simulink model "automata_learning"  (R2022a)
(part 4 of 10)

(exp(0.08277370035648346 * x1 + 0.14355190098285675 * x2 + 0.11031784117221832) - 1.0) / (exp(0.08277370035648346 * x1 + 0.14355190098285675 * x2 + 0.11031784117221832) + 1.0) - 0.17225147783756256 * (exp(0.9740955233573914 * x1 - 0.5740582346916199 * x2 + 0.584020733833313) - 1.0) / (exp(0.9740955233573914 * x1 - 0.5740582346916199 * x2 + 0.584020733833313) + 1.0) - 0.14975093305110931 * (exp(0.2844334542751312 * x1 - 0.20399335026741028 * x2 + 0.39677372574806213) - 1.0) / (exp(0.2844334542751312 * x1 - 0.20399335026741028 * x2 + 0.39677372574806213) + 1.0) - 0.6673128008842468 * (exp(0.12507730722427368 * x1 + 0.22762612998485565 * x2 + 0.3865107297897339) - 1.0) / (exp(0.12507730722427368 * x1 + 0.22762612998485565 * x2 + 0.3865107297897339) + 1.0) + 0.31276842951774597 * (exp(0.5199534296989441 * x1 - 0.738328218460083 * x2 + 0.49007365107536316) - 1.0) / (exp(0.5199534296989441 * x1 - 0.738328218460083 * x2 + 0.49007365107536316) + 1.0) - 0.4881001114845276 * (exp(0.8014535307884216 * x1 - 0.28345319628715515 * x2 + 0.22281718254089355) - 1.0) / (exp(0.8014535307884216 * x1 - 0.28345319628715515 * x2 + 0.22281718254089355) + 1.0) + 0.46977734565734863 * (exp(1.577635645866394 * x1 + 0.23506608605384827 * x2 - 0.06673777848482132) - 1.0) / (exp(1.577635645866394 * x1 + 0.23506608605384827 * x2 - 0.06673777848482132) + 1.0) + 0.3694143295288086 * (exp(0.9763611555099487 * x1 + 1.2415034770965576 * x2 - 0.16854457557201385) - 1.0) / (exp(0.9763611555099487 * x1 + 1.2415034770965576 * x2 - 0.16854457557201385) + 1.0) + 0.12421704083681107 * (exp(0.9488367438316345 * x2 - 0.4073374271392822 * x1 + 0.07838433980941772) - 1.0) / (exp(0.9488367438316345 * x2 - 0.4073374271392822 * x1 + 0.07838433980941772) + 1.0) + 0.6204631328582764 * (exp(1.727070927619934 * x1 + 0.877204418182373 * x2 + 0.7861019372940063) - 1.0) / (exp(1.727070927619934 * x1 + 0.877204418182373 * x2 + 0.7861019372940063) + 1.0) + 2.2496016025543213 * (exp(0.0031111659482121468 * x2 - 1.920979619026184 * x1 + 1.6593092679977417) - 1.0) / (exp(0.0031111659482121468 * x2 - 1.920979619026184 * x1 + 1.6593092679977417) + 1.0) + 0.0063673099502921104) + 1.0) - 0.01678931713104248 * (exp(0.025701038539409637 * (exp(0.2574288547039032 * x2 - 0.6871621012687683 * x1 + 0.5600507855415344) - 1.0) / (exp(0.2574288547039032 * x2 - 0.6871621012687683 * x1 + 0.5600507855415344) + 1.0) - 0.6211979985237122 * (exp(0.28132522106170654 * x2 - 0.539489209651947 * x1 + 0.6009179949760437) - 1.0) / (exp(0.28132522106170654 * x2 - 0.539489209651947 * x1 + 0.6009179949760437) + 1.0) - 0.07466983050107956 * (exp(0.23744763433933258 * x2 - 0.9225135445594788 * x1 + 0.3782052993774414) - 1.0) / (exp(0.23744763433933258 * x2 - 0.9225135445594788 * x1 + 0.3782052993774414) + 1.0) - 0.6362066268920898 * (exp(0.5844773054122925 * x2 - 0.2779636085033417 * x1 + 0.6274034380912781) - 1.0) / (exp(0.5844773054122925 * x2 - 0.2779636085033417 * x1 + 0.6274034380912781) + 1.0) + 0.18158797919750214 * (exp(0.18866761028766632 * x1 + 0.25410085916519165 * x2 + 0.5283621549606323) - 1.0) / (exp(0.18866761028766632 * x1 + 0.25410085916519165 * x2 + 0.5283621549606323) + 1.0) + 0.7426992654800415 * (exp(1.1490525007247925 * x1 - 0.646297037601471 * x2 + 0.6117565035820007) - 1.0) / (exp(1.1490525007247925 * x1 - 0.646297037601471 * x2 + 0.6117565035820007) + 1.0) + 0.16969242691993713 * (exp(0.20323987305164337 * x1 + 0.5146556496620178 * x2 + 0.6071406602859497) - 1.0) / (exp(0.20323987305164337 * x1 + 0.5146556496620178 * x2 + 0.6071406602859497) + 1.0) + 0.10171923041343689 * (exp(0.5478074550628662 * x1 + 0.33825451135635376 * x2 + 0.42206645011901855) - 1.0) / (exp(0.5478074550628662 * x1 + 0.33825451135635376 * x2 + 0.42206645011901855) + 1.0) - 0.7393468022346497 * (exp(1.1907950639724731 * x1 + 0.3422628939151764 * x2 - 0.10066080093383789) - 1.0) / (exp(1.1907950639724731 * x1 + 0.3422628939151764 * x2 - 0.10066080093383789) + 1.0) + 0.05626780539751053 * (exp(0.08277370035648346 * x1 + 0.14355190098285675 * x2 + 0.11031784117221832) - 1.0) / (exp(0.08277370035648346 * x1 + 0.14355190098285675 * x2 + 0.11031784117221832) + 1.0) + 0.754966676235199 * (exp(0.9740955233573914 * x1 - 0.5740582346916199 * x2 + 0.584020733833313) - 1.0) / (exp(0.9740955233573914 * x1 - 0.5740582346916199 * x2 + 0.584020733833313) + 1.0) + 0.7143430113792419 * (exp(0.2844334542751312 * x1 - 0.20399335026741028 * x2 + 0.39677372574806213) - 1.0) / (exp(0.2844334542751312 * x1 - 0.20399335026741028 * x2 + 0.39677372574806213) + 1.0) + 0.6644455790519714 * (exp(0.12507730722427368 * x1 + 0.22762612998485565 * x2 + 0.3865107297897339) - 1.0) / (exp(0.12507730722427368 * x1 + 0.22762612998485565 * x2 + 0.3865107297897339) + 1.0) - 0.20606382191181183 * (exp(0.5199534296989441 * x1 - 0.738328218460083 * x2 + 0.49007365107536316) - 1.0) / (exp(0.5199534296989441 * x1 - 0.738328218460083 * x2 + 0.49007365107536316) + 1.0) + 0.4566824436187744 * (exp(0.8014535307884216 * x1 - 0.28345319628715515 * x2 + 0.22281718254089355) - 1.0) / (exp(0.8014535307884216 * x1 - 0.28345319628715515 * x2 + 0.22281718254089355) + 1.0) - 0.7963041067123413 * (exp(1.577635645866394 * x1 + 0.23506608605384827 * x2 - 0.06673777848482132) - 1.0) / (exp(1.577635645866394 * x1 + 0.23506608605384827 * x2 - 0.06673777848482132) + 1.0) - 0.2628166675567627 * (exp(0.9763611555099487 * x1 + 1.2415034770965576 * x2 - 0.16854457557201385) - 1.0) / (exp(0.9763611555099487 * x1 + 1.2415034770965576 * x2 - 0.16854457557201385) + 1.0) + 0.245744988322258 * (exp(0.9488367438316345 * x2 - 0.4073374271392822 * x1 + 0.07838433980941772) - 1.0) / (exp(0.9488367438316345 * x2 - 0.4073374271392822 * x1 + 0.07838433980941772) + 1.0) + 0.47640275955200195 * (exp(1.727070927619934 * x1 + 0.877204418182373 * x2 + 0.7861019372940063) - 1.0) / (exp(1.727070927619934 * x1 + 0.877204418182373 * x2 + 0.7861019372940063) + 1.0) + 0.15228034555912018 * (exp(0.0031111659482121468 * x2 - 1.920979619026184 * x1 + 1.6593092679977417) - 1.0) / (exp(0.0031111659482121468 * x2 - 1.920979619026184 * x1 + 1.6593092679977417) + 1.0) + 0.0742749571800232) - 1.0) / (exp(0.025701038539409637 * (exp(0.2574288547039032 * x2 - 0.6871621012687683 * x1 + 0.5600507855415344) - 1.0) / (exp(0.2574288547039032 * x2 - 0.6871621012687683 * x1 + 0.5600507855415344) + 1.0) - 0.6211979985237122 * (exp(0.28132522106170654 * x2 - 0.539489209651947 * x1 + 0.6009179949760437) - 1.0) / (exp(0.28132522106170654 * x2 - 0.539489209651947 * x1 + 0.6009179949760437) + 1.0) - 0.07466983050107956 * (exp(0.23744763433933258 * x2 - 0.9225135445594788 * x1 + 0.3782052993774414) - 1.0) / (exp(0.23744763433933258 * x2 - 0.9225135445594788 * x1 + 0.3782052993774414) + 1.0) - 0.6362066268920898 * (exp(0.5844773054122925 * x2 - 0.2779636085033417 * x1 + 0.6274034380912781) - 1.0) / (exp(0.5844773054122925 * x2 - 0.2779636085033417 * x1 + 0.6274034380912781) + 1.0) + 0.18158797919750214 * (exp(0.18866761028766632 * x1 + 0.25410085916519165 * x2 + 0.5283621549606323) - 1.0) / (exp(0.18866761028766632 * x1 + 0.25410085916519165 * x2 + 0.5283621549606323) + 1.0) + 0.7426992654800415 * (exp(1.1490525007247925 * x1 - 0.646297037601471 * x2 + 0.6117565035820007) - 1.0) / (exp(1.1490525007247925 * x1 - 0.646297037601471 * x2 + 0.6117565035820007) + 1.0) + 0.16969242691993713 * (exp(0.20323987305164337 * x1 + 0.5146556496620178 * x2 + 0.6071406602859497) - 1.0) / (exp(0.20323987305164337 * x1 + 0.5146556496620178 * x2 + 0.6071406602859497) + 1.0) + 0.10171923041343689 * (exp(0.5478074550628662 * x1 + 0.33825451135635376 * x2 + 0.42206645011901855) - 1.0) / (exp(0.5478074550628662 * x1 + 0.33825451135635376 * x2 + 0.42206645011901855) + 1.0) - 0.7393468022346497 * (exp(1.1907950639724731 * x1 + 0.3422628939151764 * x2 - 0.10066080093383789) - 1.0) / (exp(1.1907950639724731 * x1 + 0.3422628939151764 * x2 - 0.10066080093383789) + 1.0) + 0.05626780539751053 * (exp(0.08277370035648346 * x1 + 0.14355190098285675 * x2 + 0.11031784117221832) - 1.0) / (exp(0.08277370035648346 * x1 + 0.14355190098285675 * x2 + 0.11031784117221832) + 1.0) + 0.754966676235199 * (exp(0.9740955233573914 * x1 - 0.5740582346916199 * x2 + 0.584020733833313) - 1.0) / (exp(0.9740955233573914 * x1 - 0.5740582346916199 * x2 + 0.584020733833313) + 1.0) + 0.7143430113792419 * (exp(0.2844334542751312 * x1 - 0.20399335026741028 * x2 + 0.39677372574806213) - 1.0) / (exp(0.2844334542751312 * x1 - 0.20399335026741028 * x2 + 0.39677372574806213) + 1.0) + 0.6644455790519714 * (exp(0.12507730722427368 * x1 + 0.22762612998485565 * x2 + 0.3865107297897339) - 1.0) / (exp(0.12507730722427368 * x1 + 0.22762612998485565 * x2 + 0.3865107297897339) + 1.0) - 0.20606382191181183 * (exp(0.5199534296989441 * x1 - 0.738328218460083 * x2 + 0.49007365107536316) - 1.0) / (exp(0.5199534296989441 * x1 - 0.738328218460083 * x2 + 0.49007365107536316) + 1.0) + 0.4566824436187744 * (exp(0.8014535307884216 * x1 - 0.28345319628715515 * x2 + 0.22281718254089355) - 1.0) / (exp(0.8014535307884216 * x1 - 0.28345319628715515 * x2 + 0.22281718254089355) + 1.0) - 0.7963041067123413 * (exp(1.577635645866394 * x1 + 0.23506608605384827 * x2 - 0.06673777848482132) - 1.0) / (exp(1.577635645866394 * x1 + 0.23506608605384827 * x2 - 0.06673777848482132) + 1.0) - 0.2628166675567627 * (exp(0.9763611555099487 * x1 + 1.2415034770965576 * x2 - 0.16854457557201385) - 1.0) / (exp(0.9763611555099487 * x1 + 1.2415034770965576 * x2 - 0.16854457557201385) + 1.0) + 0.245744988322258 * (exp(0.9488367438316345 * x2 - 0.4073374271392822 * x1 + 0.07838433980941772) - 1.0) / (exp(0.9488367438316345 * x2 - 0.4073374271392822 * x1 + 0.07838433980941772) + 1.0) + 0.47640275955200195 * (exp(1.727070927619934 * x1 + 0.877204418182373 * x2 + 0.7861019372940063) - 1.0) / (exp(1.727070927619934 * x1 + 0.877204418182373 * x2 + 0.7861019372940063) + 1.0) + 0.15228034555912018 * (exp(0.0031111659482121468 * x2 - 1.920979619026184 * x1 + 1.6593092679977417) - 1.0) / (exp(0.0031111659482121468 * x2 - 1.920979619026184 * x1 + 1.6593092679977417) + 1.0) + 0.0742749571800232) + 1.0) + 0.015218996442854404 * (exp(0.46923908591270447 * (exp(0.23744763433933258 * x2 - 0.9225135445594788 * x1 + 0.3782052993774414) - 1.0) / (exp(0.23744763433933258 * x2 - 0.9225135445594788 * x1 + 0.3782052993774414) + 1.0) + 0.2346094697713852 * (exp(0.28132522106170654 * x2 - 0.539489209651947 * x1 + 0.6009179949760437) - 1.0) / (exp(0.28132522106170654 * x2 - 0.539489209651947 * x1 + 0.6009179949760437) + 1.0) - 0.3579394817352295 * (exp(0.2574288547039032 * x2 - 0.6871621012687683 * x1 + 0.5600507855415344) - 1.0) / (exp(0.2574288547039032 * x2 - 0.6871621012687683 * x1 + 0.5600507855415344) + 1.0) - 0.00037727123708464205 * (exp(0.5844773054122925 * x2 - 0.2779636085033417 * x1 + 0.6274034380912781) - 1.0) / (exp(0.5844773054122925 * x2 - 0.2779636085033417 * x1 + 0.6274034380912781) + 1.0) + 0.1678800731897354 * (exp(0.18866761028766632 * x1 + 0.25410085916519165 * x2 + 0.5283621549606323) - 1.0) / (exp(0.18866761028766632 * x1 + 0.25410085916519165 * x2 + 0.5283621549606323) + 1.0) + 0.0013105710968375206 * (exp(1.1490525007247925 * x1 - 0.646297037601471 * x2 + 0.6117565035820007) - 1.0) / (exp(1.1490525007247925 * x1 - 0.646297037601471 * x2 + 0.6117565035820007) + 1.0) - 0.2674686014652252 * (exp(0.20323987305164337 * x1 + 0.5146556496620178 * x2 + 0.6071406602859497) - 1.0) / (exp(0.20323987305164337 * x1 + 0.5146556496620178 * x2 + 0.6071406602859497) + 1.0) - 0.2200189083814621 * (exp(0.5478074550628662 * x1 + 0.33825451135635376 * x2 + 0.42206645011901855) - 1.0) / (exp(0.5478074550628662 * x1 + 0.33825451135635376 * x2 + 0.42206645011901855) + 1.0) - 0.20613259077072144 * (exp(1.1907950639724731 * x1 + 0.3422628939151764 * x2 - 0.10066080093383789) - 1.0) / (exp(1.1907950639724731 * x1 + 0.3422628939151764 * x2 - 0.10066080093383789) + 1.0) + 0.3182278573513031 * (exp(0.08277370035648346 * x1 + 0.14355190098285675 * x2 + 0.11031784117221832) - 1.0) / (exp(0.08277370035648346 * x1 + 0.14355190098285675 * x2 + 0.11031784117221832) + 1.0) + 0.6413242220878601 * (exp(0.9740955233573914 * x1 - 0.5740582346916199 * x2 + 0.584020733833313) - 1.0) / (exp(0.9740955233573914 * x1 - 0.5740582346916199 * x2 + 0.584020733833313) + 1.0) + 0.09479638189077377 * (exp(0.2844334542751312 * x1 - 0.20399335026741028 * x2 + 0.39677372574806213) - 1.0) / (exp(0.2844334542751312 * x1 - 0.20399335026741028 * x2 + 0.39677372574806213) + 1.0) - 0.057093001902103424 * (exp(0.12507730722427368 * x1 + 0.22762612998485565 * x2 + 0.3865107297897339) - 1.0) / (exp(0.12507730722427368 * x1 + 0.22762612998485565 * x2 + 0.3865107297897339) + 1.0) + 0.43237894773483276 * (exp(0.5199534296989441 * x1 - 0.738328218460083 * x2 + 0.49007365107536316) - 1.0) / (exp(0.5199534296989441 * x1 - 0.738328218460083 * x2 + 0.49007365107536316) + 1.0) - 0.23227927088737488 * (exp(0.8014535307884216 * x1 - 0.28345319628715515 * x2 + 0.22281718254089355) - 1.0) / (exp(0.8014535307884216 * x1 - 0.28345319628715515 * x2 + 0.22281718254089355) + 1.0) - 0.2612578868865967 * (exp(1.577635645866394 * x1 + 0.23506608605384827 * x2 - 0.06673777848482132) - 1.0) / (exp(1.577635645866394 * x1 + 0.23506608605384827 * x2 - 0.06673777848482132) + 1.0) - 0.35415515303611755 * (exp(0.9763611555099487 * x1 + 1.2415034770965576 * x2 - 0.16854457557201385) - 1.0) / (exp(0.9763611555099487 * x1 + 1.2415034770965576 * x2 - 0.16854457557201385) + 1.0) + 0.7701698541641235 * (exp(0.9488367438316345 * x2 - 0.4073374271392822 * x1 + 0.07838433980941772) - 1.0) / (exp(0.9488367438316345 * x2 - 0.4073374271392822 * x1 + 0.07838433980941772) + 1.0) + 0.5897926092147827 * (exp(1.727070927619934 * x1 + 0.877204418182373 * x2 + 0.7861019372940063) - 1.0) / (exp(1.727070927619934 * x1 + 0.877204418182373 * x2 + 0.7861019372940063) + 1.0) + 0.2892034947872162 * (exp(0.0031111659482121468 * x2 - 1.920979619026184 * x1 + 1.6593092679977417) - 1.0) / (exp(0.0031111659482121468 * x2 - 1.920979619026184 * x1 + 1.6593092679977417) + 1.0) + 0.04858407750725746) - 1.0) / (exp(0.46923908591270447 * (exp(0.23744763433933258 * x2 - 0.9225135445594788 * x1 + 0.3782052993774414) - 1.0) / (exp(0.23744763433933258 * x2 - 0.9225135445594788 * x1 + 0.3782052993774414) + 1.0) + 0.2346094697713852 * (exp(0.28132522106170654 * x2 - 0.539489209651947 * x1 + 0.6009179949760437) - 1.0) / (exp(0.28132522106170654 * x2 - 0.539489209651947 * x1 + 0.6009179949760437) + 1.0) - 0.3579394817352295 * (exp(0.2574288547039032 * x2 - 0.6871621012687683 * x1 + 0.5600507855415344) - 1.0) / (exp(0.2574288547039032 * x2 - 0.6871621012687683 * x1 + 0.5600507855415344) + 1.0) - 0.00037727123708464205 * (exp(0.5844773054122925 * x2 - 0.2779636085033417 * x1 + 0.6274034380912781) - 1.0) / (exp(0.5844773054122925 * x2 - 0.2779636085033417 * x1 + 0.6274034380912781) + 1.0) + 0.1678800731897354 * (exp(0.18866761028766632 * x1 + 0.25410085916519165 * x2 + 0.5283621549606323) - 1.0) / (exp(0.18866761028766632 * x1 + 0.25410085916519165 * x2 + 0.5283621549606323) + 1.0) + 0.0013105710968375206 * (exp(1.1490525007247925 * x1 - 0.646297037601471 * x2 + 0.6117565035820007) - 1.0) / (exp(1.1490525007247925 * x1 - 0.646297037601471 * x2 + 0.6117565035820007) + 1.0) - 0.2674686014652252 * (exp(0.20323987305164337 * x1 + 0.5146556496620178 * x2 + 0.6071406602859497) - 1.0) / (exp(0.20323987305164337 * x1 + 0.5146556496620178 * x2 + 0.6071406602859497) + 1.0) - 0.2200189083814621 * (exp(0.5478074550628662 * x1 + 0.33825451135635376 * x2 + 0.42206645011901855) - 1.0) / (exp(0.5478074550628662 * x1 + 0.33825451135635376 * x2 + 0.42206645011901855) + 1.0) - 0.20613259077072144 * (exp(1.1907950639724731 * x1 + 0.3422628939151764 * x2 - 0.10066080093383789) - 1.0) / (exp(1.1907950639724731 * x1 + 0.3422628939151764 * x2 - 0.10066080093383789) + 1.0) + 0.3182278573513031 * (exp(0.08277370035648346 * x1 + 0.14355190098285675 * x2 + 0.11031784117221832) - 1.0) / (exp(0.08277370035648346 * x1 + 0.14355190098285675 * x2 + 0.11031784117221832) + 1.0) + 0.6413242220878601 * (exp(0.9740955233573914 * x1 - 0.5740582346916199 * x2 + 0.584020733833313) - 1.0) / (exp(0.9740955233573914 * x1 - 0.5740582346916199 * x2 + 0.584020733833313) + 1.0) + 0.09479638189077377 * (exp(0.2844334542751312 * x1 - 0.20399335026741028 * x2 + 0.39677372574806213) - 1.0) / (exp(0.2844334542751312 * x1 - 0.20399335026741028 * x2 + 0.39677372574806213) + 1.0) - 0.057093001902103424 * (exp(0.12507730722427368 * x1 + 0.22762612998485565 * x2 + 0.3865107297897339) - 1.0) / (exp(0.12507730722427368 * x1 + 0.22762612998485565 * x2 + 0.3865107297897339) + 1.0) + 0.43237894773483276 * (exp(0.5199534296989441 * x1 - 0.738328218460083 * x2 + 0.49007365107536316) - 1.0) / (exp(0.5199534296989441 * x1 - 0.738328218460083 * x2 + 0.49007365107536316) + 1.0) - 0.23227927088737488 * (exp(0.8014535307884216 * x1 - 0.28345319628715515 * x2 + 0.22281718254089355) - 1.0) / (exp(0.8014535307884216 * x1 - 0.28345319628715515 * x2 + 0.22281718254089355) + 1.0) - 0.2612578868865967 * (exp(1.577635645866394 * x1 + 0.23506608605384827 * x2 - 0.06673777848482132) - 1.0) / (exp(1.577635645866394 * x1 + 0.23506608605384827 * x2 - 0.06673777848482132) + 1.0) - 0.35415515303611755 * (exp(0.9763611555099487 * x1 + 1.2415034770965576 * x2 - 0.16854457557201385) - 1.0) / (exp(0.9763611555099487 * x1 + 1.2415034770965576 * x2 - 0.16854457557201385) + 1.0) + 0.7701698541641235 * (exp(0.9488367438316345 * x2 - 0.4073374271392822 * x1 + 0.07838433980941772) - 1.0) / (exp(0.9488367438316345 * x2 - 0.4073374271392822 * x1 + 0.07838433980941772) + 1.0) + 0.5897926092147827 * (exp(1.727070927619934 * x1 + 0.877204418182373 * x2 + 0.7861019372940063) - 1.0) / (exp(1.727070927619934 * x1 + 0.877204418182373 * x2 + 0.7861019372940063) + 1.0) + 0.2892034947872162 * (exp(0.0031111659482121468 * x2 - 1.920979619026184 * x1 + 1.6593092679977417) - 1.0) / (exp(0.0031111659482121468 * x2 - 1.920979619026184 * x1 + 1.6593092679977417) + 1.0) + 0.04858407750725746) + 1.0) + 0.05119678005576134;
